simulink model "chauffage_barre_3"  (R2019b)
settings: Solver=VariableStepAuto  StartTime=0.0  StopTime=3600*2  RelTol=1e-3
libraries: fl_lib x10, nesl_utility x5
settings Model: Creator=Ivan  LastModifiedBy=ivanl

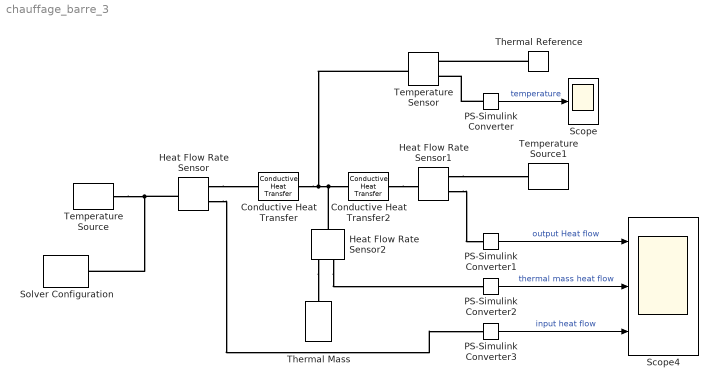
== system chauffage_barre_3 ==
  Conductive Heat Transfer : fl_lib/Thermal/Thermal Elements/Conductive Heat Transfer  area=8 cm^2  thickness=10 cm  th_cond=50 W/(m*K)  T_specify=off  T_priority=None  T=0 K  T_nominal_specify=off  T_nominal_unit=K  T_nominal_value=1  Q_specify=off  Q_priority=None  Q=0 W  Q_nominal_specify=off  Q_nominal_unit=W  Q_nominal_value=1
      settings: SourceProductName=Simscape
  Conductive Heat Transfer2 : fl_lib/Thermal/Thermal Elements/Conductive Heat Transfer  area=8 cm^2  thickness=10 cm  th_cond=50 W/(m*K)  T_specify=off  T_priority=None  T=0 K  T_nominal_specify=off  T_nominal_unit=K  T_nominal_value=1  Q_specify=off  Q_priority=None  Q=0 W  Q_nominal_specify=off  Q_nominal_unit=W  Q_nominal_value=1
      settings: SourceProductName=Simscape
  Heat Flow Rate Sensor : fl_lib/Thermal/Thermal Sensors/Heat Flow Rate Sensor
      settings: SourceProductName=Simscape  SourceProductBaseCode=SS
  Heat Flow Rate Sensor1 : fl_lib/Thermal/Thermal Sensors/Heat Flow Rate Sensor
      settings: SourceProductName=Simscape  SourceProductBaseCode=SS
  Heat Flow Rate Sensor2 : fl_lib/Thermal/Thermal Sensors/Heat Flow Rate Sensor
      settings: SourceProductName=Simscape  SourceProductBaseCode=SS
  PS-Simulink Converter : nesl_utility/PS-Simulink Converter  PhysicalDomain=network_engine_domain  SubClassName=ps_output  LeftPortType=input  RightPortType=output  PseudoPeriodic=off  Frequencies=[]  Unit=degC  AffineConversion=on
  PS-Simulink Converter1 : nesl_utility/PS-Simulink Converter  PhysicalDomain=network_engine_domain  SubClassName=ps_output  LeftPortType=input  RightPortType=output  PseudoPeriodic=off  Frequencies=[]  Unit=W  AffineConversion=on
  PS-Simulink Converter2 : nesl_utility/PS-Simulink Converter  PhysicalDomain=network_engine_domain  SubClassName=ps_output  LeftPortType=input  RightPortType=output  PseudoPeriodic=off  Frequencies=[]  Unit=W  AffineConversion=on
  PS-Simulink Converter3 : nesl_utility/PS-Simulink Converter  PhysicalDomain=network_engine_domain  SubClassName=ps_output  LeftPortType=input  RightPortType=output  PseudoPeriodic=off  Frequencies=[]  Unit=J/s  AffineConversion=on
  Scope : Scope
  Scope4 : Scope  NumInputPorts=3
  Solver Configuration : nesl_utility/Solver Configuration  PhysicalDomain=network_engine_domain  SubClassName=solver  LeftPortType=input  RightPortType=generic  Tones=[]  Harmonics=[]  SimulateNoise=off  Profile=off  UseLocalSampling=off  EnableSwitchedLinearOptims=on  FrequencyDomain=off  UseCCode=off  RelTol=0.001  AbsTol=1e-06  MinStep=1e-09  ToWorkspace=off  RevertToSquareIcSolve=off  NumHomotopyIterations=100  PhasorMode=off  PhasorModeNumHarmonics=1  DoDC=off  ResidualTolerance=1e-09  UseLocalSolver=off  LocalSolverChoice=NE_BACKWARD_EULER_ADVANCER  LocalSolverSampleTime=0.001  DoFixedCost=off  MaxNonlinIter=3  MaxModeIter=2  LinearAlgebra=auto  EquationFormulation=NE_TIME_EF  DelaysMemoryBudget=1024  AutomaticFiltering=on  FilteringTimeConstant=0.001  PartitionStorageMethod=AS_NEEDED  PartitionMemoryBudget=1024  PartitionMethod=ROBUST
  Temperature Sensor : fl_lib/Thermal/Thermal Sensors/Temperature Sensor
  Temperature Source : fl_lib/Thermal/Thermal Sources/Temperature Source  temperature=300 degC
      settings: SourceProductName=Simscape
  Temperature Source1 : fl_lib/Thermal/Thermal Sources/Temperature Source  temperature=0 degC
      settings: SourceProductName=Simscape
  Thermal Mass : fl_lib/Thermal/Thermal Elements/Thermal Mass  mass=1.248 kg  sp_heat=444 J/kg/K  T_specify=on  T_priority=High  T=20 degC  T_nominal_specify=off  T_nominal_unit=K  T_nominal_value=1  Q_specify=off  Q_priority=None  Q=0 W  Q_nominal_specify=off  Q_nominal_unit=W  Q_nominal_value=1
  Thermal Reference : fl_lib/Thermal/Thermal Elements/Thermal Reference
  wires:
  PS-Simulink Converter/1 -> Scope/1  "temperature"
  PS-Simulink Converter1/1 -> Scope4/1  "output Heat flow"
  PS-Simulink Converter2/1 -> Scope4/2  "thermal mass heat flow"
  PS-Simulink Converter3/1 -> Scope4/3  "input heat flow"
  connections:
  Conductive Heat Transfer/RConn1 -- Temperature Sensor/LConn1 -- Conductive Heat Transfer2/LConn1 -- Heat Flow Rate Sensor2/LConn1
  Temperature Source/LConn1 -- Heat Flow Rate Sensor/LConn1 -- Solver Configuration/RConn1
  Thermal Reference/LConn1 -- Temperature Sensor/RConn1
  PS-Simulink Converter/LConn1 -- Temperature Sensor/RConn2
  Heat Flow Rate Sensor/RConn2 -- Conductive Heat Transfer/LConn1
  Heat Flow Rate Sensor2/RConn2 -- Thermal Mass/LConn1
  Conductive Heat Transfer2/RConn1 -- Heat Flow Rate Sensor1/LConn1
  Heat Flow Rate Sensor1/RConn2 -- Temperature Source1/LConn1
  Heat Flow Rate Sensor/RConn1 -- PS-Simulink Converter3/LConn1
  Heat Flow Rate Sensor2/RConn1 -- PS-Simulink Converter2/LConn1
  Heat Flow Rate Sensor1/RConn1 -- PS-Simulink Converter1/LConn1
